simulink model "HBsimRL_closed"  (R2018b)
settings: Solver=ode4  StartTime=0.0  StopTime=0.5e-3*0+0.015  FixedStep=Tsim  MaxStep=1e-4  RelTol=1e-6
values from neighbouring files (symbols this model uses):
  fsw = PWM_frequency    (= 10000)    [closedRL_init.m]
  ki = wc*Req    (= 20850)    [closedRL_init.m]
  kp = wc*L    (= 2.58)    [closedRL_init.m]
  L = 860e-6    (= 0.00086)    [closedRL_init.m]
  Rl = 0.15    [closedRL_init.m]
  Ro = 6.8    [closedRL_init.m]
  Ts = Tsw    (= 0.0001)    [closedRL_init.m]
  Tsim = Tsw/400    (= 2.5e-07)    [closedRL_init.m]
  Vdc = 15    [closedRL_init.m]
libraries: powerlib x8, simulink x4
settings Model: Creator=matti  LastModifiedBy=matti
settings DataIOCC: ReturnWorkspaceOutputs=on

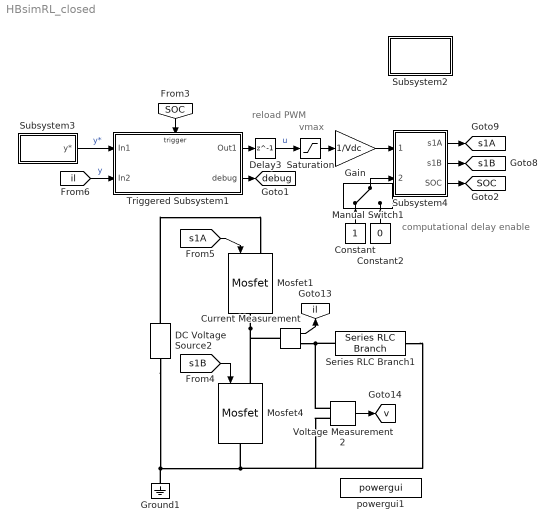
== system HBsimRL_closed ==
  note: reload
      | PWM
  note: computational delay
      | enable
  note: vmax
  Constant : Constant  SampleTime=Ts
  Constant2 : Constant  Value=0  SampleTime=Ts
  Current Measurement : powerlib/Measurements/Current Measurement  PhasorSimulation=off  OutputType=Complex  PSBequivalent=0
  DC Voltage Source2 : powerlib/Electrical Sources/DC Voltage Source  Amplitude=Vdc  Measurements=None
      settings: SourceProductName=Simscape Electrical
  Delay3 : Delay  DelayLength=1  SampleTime=Ts/2
  Gain : Gain  Gain=1/Vdc
  Ground1 : powerlib/Elements/Ground  LConnTagsString=a
      settings: SourceProductName=Simscape Electrical
  Manual Switch1 : ManualSwitch
  Mosfet1 : powerlib/Power Electronics/Mosfet  Ron=0.1  Lon=0  Rd=0.01  Vfd=0  IC=0  Rs=1e5  Cs=inf  Measurements=off
      settings: SourceProductName=Simscape Electrical
  Mosfet4 : powerlib/Power Electronics/Mosfet  Ron=0.1  Lon=0  Rd=0.01  Vfd=0  IC=0  Rs=1e5  Cs=inf  Measurements=off
      settings: SourceProductName=Simscape Electrical
  Saturation : Saturate  UpperLimit=Vdc*0.98  LowerLimit=0
  Series RLC Branch1 : powerlib/Elements/Series RLC Branch  LConnTagsString=__new0  RConnTagsString=__new0  BranchType=RL  Resistance=Ro+Rl  Inductance=L  SetiL0=off  InitialCurrent=0.1  Capacitance=1e-6  Setx0=off  InitialVoltage=0  Measurements=None
  Subsystem2 : Subsystem
      mask Display: disp('stream')
  Subsystem3 : Subsystem
      mask Display: disp('reference')
  Subsystem4 : Subsystem
      mask Display: disp('modulator')
  Triggered Subsystem1 : Subsystem  TreatAsAtomicUnit=on
      mask Display: disp('current controller\n(syncronized with PWM)')
  Voltage Measurement2 : powerlib/Measurements/Voltage Measurement  PhasorSimulation=off  OutputType=Complex  PSBequivalent=0
  powergui1 : powerlib/powergui  Priority=1  SimulationMode=Continuous  SampleTime=1/(400*fsw)  frequency=60  Iterations=50  frequencyindice=0  Pbase=100e6  ErrMax=1e-4  UnitsV=kV  UnitsW=MW  buscounter=0  FunctionMessages=off  echomessages=off  EnableUseOfTLC=off  CurrentSourceSwitches=off  DisableSnubberDevices=on  DisableRonSwitches=on  DisableVfSwitches=on  DisplayEquations=off  SolverType=Tustin/Backward Euler (TBE)  Interpol=off  ExternalGateDelay=off  methode=off  Ts=100  x0status=blocks  SPID=off  SwTol=0  HookPort=off  RestoreLinks=warning  ResistiveCurrentMeasurement=off  Frange=[0:2:500]  Ylog=off  Xlog=on  ShowGrid=off  save=off  variable=ZData  structure=0  ZoomFFT=off  StartTime=0.0  cycles=1  DisplayStyle=1  fundamental=60  FreqAxis=off  MaxFrequency=1000  frequencyindicesteady=1  RmsSteady=1  display=off
  tag scope: SOC=global, debug=global, il=global, s1A=global, s1B=global, v=global
  wires:
  Current Measurement/1 -> [il]
  Voltage Measurement2/1 -> [v]
  Saturation/1 -> Gain/1
  Gain/1 -> Subsystem4/1(modA)
  [s1A] -> Mosfet1/1
  [s1B] -> Mosfet4/1
  Subsystem4/1(s1A) -> [s1A]
  Subsystem4/2(s1B) -> [s1B]
  Manual Switch1/1 -> Subsystem4/2(enable delay)
  Constant/1 -> Manual Switch1/1
  Constant2/1 -> Manual Switch1/2
  Subsystem4/3(SOC) -> [SOC]
  Triggered Subsystem1/1(Out1) -> Delay3/1
  [SOC] -> Triggered Subsystem1/Trigger
  Triggered Subsystem1/2(debug) -> [debug]
  Subsystem3/1(y*) -> Triggered Subsystem1/1(In1)  "y*"
  [il] -> Triggered Subsystem1/2(In2)  "y"
  Delay3/1 -> Saturation/1  "u"
  connections:
  Mosfet1/RConn1 -- Current Measurement/LConn1 -- Mosfet4/LConn1
  DC Voltage Source2/RConn1 -- Mosfet1/LConn1
  Voltage Measurement2/LConn1 -- Current Measurement/RConn1 -- Series RLC Branch1/LConn1
  DC Voltage Source2/LConn1 -- Ground1/LConn1 -- Series RLC Branch1/RConn1 -- Voltage Measurement2/LConn2 -- Mosfet4/RConn1

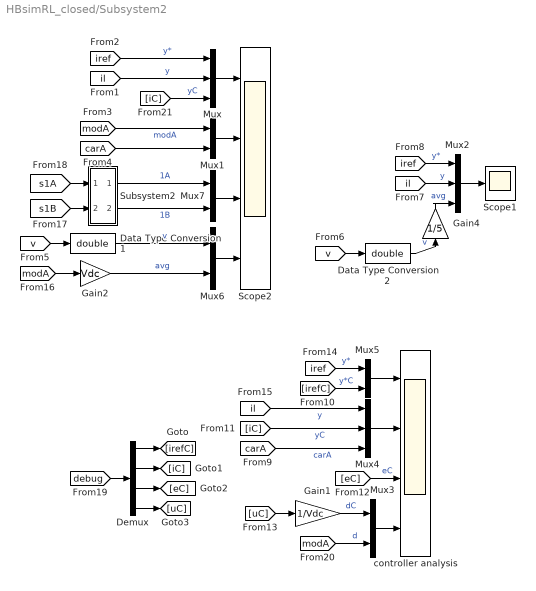
== system HBsimRL_closed/Subsystem2 ==
  Data Type Conversion1 : DataTypeConversion  OutDataTypeStr=double
  Data Type Conversion2 : DataTypeConversion  OutDataTypeStr=double
  Demux : Demux
  Gain1 : Gain  Gain=1/Vdc
  Gain2 : Gain  Gain=Vdc
  Gain4 : Gain  Gain=1/5
  Mux : Mux  Inputs=3
  Mux{1,3,5..7} (5 alike) : Mux  Inputs=2
  Mux2 : Mux  Inputs=3
  Mux4 : Mux  Inputs=3
  Scope1 : Scope
  Scope2 : Scope  NumInputPorts=4
  Subsystem2 : Subsystem
      mask Display: disp('shift')
  controller analysis : Scope  NumInputPorts=4
  wires:
  Mux1/1 -> Scope2/2
  Data Type Conversion1/1 -> Mux6/1  "v"
  [modA] -> Gain2/1
  Mux6/1 -> Scope2/4
  [carA] -> Mux1/2
  [v] -> Data Type Conversion1/1
  [s1B] -> Subsystem2/2(In2)
  Gain2/1 -> Mux6/2  "avg"
  Subsystem2/1(Out1) -> Mux7/1  "1A"
  Mux7/1 -> Scope2/3
  [modA] -> Mux1/1  "modA"
  Subsystem2/2(Out2) -> Mux7/2  "1B"
  [s1A] -> Subsystem2/1(In1)
  [v] -> Data Type Conversion2/1
  Data Type Conversion2/1 -> Gain4/1  "v"
  [iref] -> Mux2/1  "y*"
  [il] -> Mux2/2  "y"
  Mux2/1 -> Scope1/1
  Gain4/1 -> Mux2/3  "avg"
  [iref] -> Mux/1  "y*"
  [il] -> Mux/2  "y"
  Mux/1 -> Scope2/1
  [eC] -> controller analysis/3  "eC"
  Mux3/1 -> controller analysis/4
  Mux5/1 -> controller analysis/1
  Mux4/1 -> controller analysis/2
  [iref] -> Mux5/1  "y*"
  [uC] -> Gain1/1
  [il] -> Mux4/1  "y"
  [iC] -> Mux4/2  "yC"
  [carA] -> Mux4/3  "carA"
  [modA] -> Mux3/2  "d"
  [debug] -> Demux/1
  Demux/3 -> [eC]
  Demux/2 -> [iC]
  Demux/1 -> [irefC]
  Demux/4 -> [uC]
  [irefC] -> Mux5/2  "y*C"
  Gain1/1 -> Mux3/1  "dC"
  [iC] -> Mux/3  "yC"

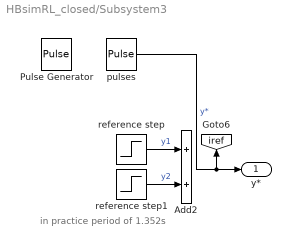
== system HBsimRL_closed/Subsystem3 ==
  note: in practice period of 1.352s
  Add2 : Sum
  Pulse Generator : DiscretePulseGenerator  PulseType=Time based  Amplitude=6  Period=3  PulseWidth=50
  pulses : DiscretePulseGenerator  Amplitude=1.5  Period=120  PulseWidth=60  PhaseDelay=5  SampleTime=Ts
  reference step : Step  Time=2e-3  After=1.8  SampleTime=Ts
  reference step1 : Step  Time=0.01  After=-1.8  SampleTime=Ts
  y* : Outport
  tag scope: iref=global
  wires:
  reference step1/1 -> Add2/2  "y2"
  pulses/1 -> [iref], y*/1  "y*"
  reference step/1 -> Add2/1  "y1"

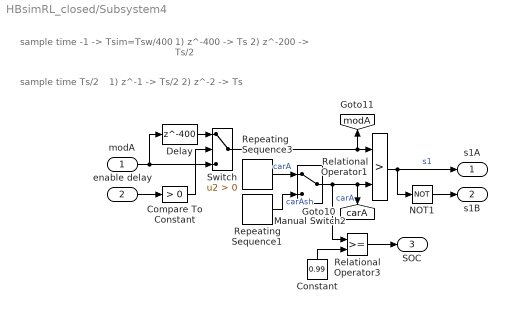
== system HBsimRL_closed/Subsystem4 ==
  note: sample time Ts/2
  note: 1)  z^-1 -> Ts/2
      | 2)  z^-2 -> Ts
  note: sample time -1 -> Tsim=Tsw/400
  note: 1)  z^-400 -> Ts
      | 2)  z^-200 -> Ts/2
  modA : Inport
  enable delay : Inport  Port=2
  Compare To Constant : simulink/Logic and Bit Operations/Compare To Constant  relop=>  const=0  OutDataTypeStr=boolean
  Constant : Constant  Value=0.99  SampleTime=Ts
  Delay : Delay  DelayLength=400  SampleTime=Tsim
  Manual Switch2 : ManualSwitch
  NOT1 : Logic  Operator=NOT  IconShape=distinctive  AllPortsSameDT=off  OutDataTypeStr=boolean
  Relational Operator1 : RelationalOperator  Operator=>  OutDataTypeStr=boolean  RndMeth=Simplest
  Relational Operator3 : RelationalOperator  OutDataTypeStr=boolean  RndMeth=Simplest
  Repeating Sequence1 : simulink/Sources/Repeating Sequence  rep_seq_t=[0 1/(4*fsw) 1/(2*fsw) 3/(4*fsw) 1/fsw]  rep_seq_y=[0.5 0 0.5 1 0.5]
  Repeating Sequence3 : simulink/Sources/Repeating Sequence  rep_seq_t=[0 1/(2*fsw) 1/fsw]  rep_seq_y=[0 1 0]
  Switch : Switch  Criteria=u2 > Threshold
  s1A : Outport
  s1B : Outport  Port=2
  SOC : Outport  Port=3
  tag scope: carA=global, modA=global
  wires:
  Switch/1 -> [modA], Relational Operator1/1
  Manual Switch2/1 -> Relational Operator3/1, [carA], Relational Operator1/2  "carA"
  Relational Operator1/1 -> NOT1/1, s1A/1  "s1"
  Repeating Sequence1/1 -> Manual Switch2/2  "carAsh"
  Repeating Sequence3/1 -> Manual Switch2/1  "carA"
  NOT1/1 -> s1B/1
  Constant/1 -> Relational Operator3/2
  Delay/1 -> Switch/1
  Compare To Constant/1 -> Switch/2
  modA/1 -> Delay/1, Switch/3
  enable delay/1 -> Compare To Constant/1
  Relational Operator3/1 -> SOC/1

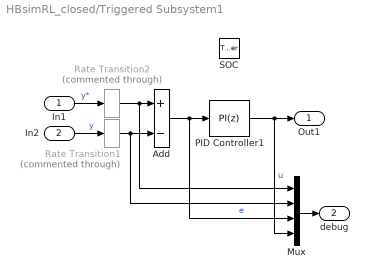
== system HBsimRL_closed/Triggered Subsystem1 ==
  In1 : Inport
  In2 : Inport  Port=2
  SOC : TriggerPort  VariantControl=Variant
  Add : Sum  Inputs=+-
  Mux : Mux
  PID Controller1 : simulink/Continuous/PID Controller  Controller=PI  Form=Parallel  TimeDomain=Discrete-time  SampleTime=-1  IntegratorMethod=Backward Euler  FilterMethod=Forward Euler  ControllerParametersSource=internal  P=kp  I=ki  D=0  UseFilter=on  N=100  TunerSelectOption=Transfer Function Based (PID Tuner App)  InitialConditionSource=internal  InitialConditionForIntegrator=0  InitialConditionForFilter=0  DifferentiatorICPrevScaledInput=0  ExternalReset=none  TrackingMode=off  Kt=1  LimitOutput=off  UpperSaturationLimit=Vdc*0.98  LowerSaturationLimit=0  LinearizeAsGain=on  AntiWindupMode=back-calculation  Kb=ki/kp  POutMin=[]  POutMax=[]  IOutMin=[]  IOutMax=[]  DOutMin=[]  DOutMax=[]  NOutMin=[]  NOutMax=[]  SumOutMin=[]  SumOutMax=[]  SaturationOutMin=[]  SaturationOutMax=[]  PParamMin=[]  PParamMax=[]  IParamMin=[]  IParamMax=[]  DParamMin=[]  DParamMax=[]  NParamMin=[]  NParamMax=[]  KbParamMin=[]  KbParamMax=[]  KtParamMin=[]  KtParamMax=[]  KbOutMin=[]  KbOutMax=[]  KtOutMin=[]  KtOutMax=[]  IntegratorOutMin=[]  IntegratorOutMax=[]  FilterOutMin=[]  FilterOutMax=[]  SumI1OutMin=[]  SumI1OutMax=[]  SumI2OutMin=[]  SumI2OutMax=[]  SumI3OutMin=[]  SumI3OutMax=[]  SumI4OutMin=[]  SumI4OutMax=[]  SumDOutMin=[]  SumDOutMax=[]  DifferentiatorOutMin=[]  DifferentiatorOutMax=[]  FilterDiffOutCoefMin=[]  FilterDiffOutCoefMax=[]  ReciprocalOutMin=[]  ReciprocalOutMax=[]  SumDenOutMin=[]  SumDenOutMax=[]  SumNumOutMin=[]  SumNumOutMax=[]  DivideOutMin=[]  DivideOutMax=[]  IntegratorContinuousStateAttributes=''  IntegratorStateMustResolveToSignalObject=off  IntegratorRTWStateStorageClass=Auto  FilterContinuousStateAttributes=''  FilterStateMustResolveToSignalObject=off  FilterRTWStateStorageClass=Auto  ParallelPVariant=InternalParameters  IdealPVariant=Disabled  IVariant=InternalParameters  DVariant=Disabled  IntegratorVariant=Discrete  SatVariant=Disabled  AWVariant=Passthrough  PCopyVariant=Disabled  TRVariant=Disabled  FdbkBlocksVariant=Forward  IdealPFdbkVariant=Disabled  SatFdbkVariant=Disabled  DerivativeFilterVariant=Disabled  NVariant=Disabled  NCopyVariant=Disabled_SignalSpec  FilterICVariant=Disabled  IntegratorICVariant=InternalICs  ExternalResetVariant=Disabled  TRSumVariant=Passthrough  SumFdbkVariant=Disabled  SumVariant=Sum_PI
  Rate Transition1 : RateTransition  Commented=through  OutPortSampleTime=Ts
  Rate Transition2 : RateTransition  Commented=through  OutPortSampleTime=Ts
  Out1 : Outport
  debug : Outport  Port=2
  wires:
  In2/1 -> Rate Transition1/1  "y"
  Add/1 -> Mux/3, PID Controller1/1  "e"
  Rate Transition2/1 -> Mux/1, Add/1
  In1/1 -> Rate Transition2/1  "y*"
  PID Controller1/1 -> Out1/1, Mux/4  "u"
  Rate Transition1/1 -> Add/2, Mux/2
  Mux/1 -> debug/1

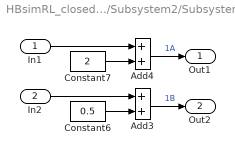
== system HBsimRL_closed/Subsystem2/Subsystem2 ==
  In1 : Inport
  In2 : Inport  Port=2
  Add3 : Sum
  Add4 : Sum
  Constant6 : Constant  Value=0.5  SampleTime=1/(200*fsw)
  Constant7 : Constant  Value=2  SampleTime=1/(200*fsw)
  Out1 : Outport
  Out2 : Outport  Port=2
  wires:
  In2/1 -> Add3/1
  In1/1 -> Add4/1
  Constant6/1 -> Add3/2
  Constant7/1 -> Add4/2
  Add4/1 -> Out1/1  "1A"
  Add3/1 -> Out2/1  "1B"
